simulink model "PID"  (R2018b)
settings: Solver=ode4  StartTime=0.0  StopTime=100  FixedStep=0.002  RelTol=1e-3
undefined symbols (not defined in the file): delta_mais, delta_menos, Kd, Ki, Km, Kp, tau
settings Model: Creator=pedro  LastModifiedBy=pedro
settings SFSimCC: SimUseLocalCustomCode=off
settings RTWCC: RTWUseLocalCustomCode=off
settings CodeAppCC: StateflowObjectComments=on

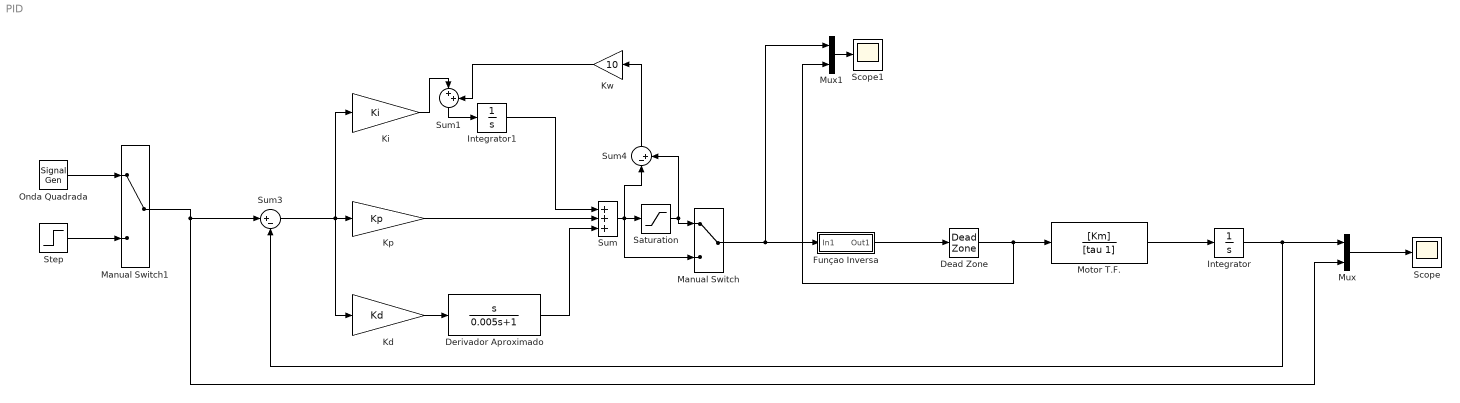
== system PID ==
  Dead Zone : DeadZone  LowerValue=-0.1154  UpperValue=0.2029  SaturateOnIntegerOverflow=on
  Derivador Aproximado : TransferFcn  Numerator=[1 0]  Denominator=[0.005 1]
  Funçao Inversa : Subsystem
  Integrator : Integrator
  Integrator1 : Integrator
  Kd : Gain  Gain=Kd
  Ki : Gain  Gain=Ki
  Kp : Gain  Gain=Kp
  Kw : Gain  Gain=10
  Manual Switch : ManualSwitch
  Manual Switch1 : ManualSwitch
  Motor T.F. : TransferFcn  Numerator=[Km]  Denominator=[tau 1]
  Mux : Mux  Inputs=2
  Mux1 : Mux  Inputs=2
  Onda Quadrada : SignalGenerator  WaveForm=square  Amplitude=20  Units=rad/sec
  Saturation : Saturate  UpperLimit=7.2  LowerLimit=-7.2
  Scope : Scope
  Scope1 : Scope
  Step : Step  SampleTime=0
  Sum : Sum  Inputs=|+|+|+|
  Sum1 : Sum  Inputs=|++
  Sum3 : Sum  Inputs=|+-
  Sum4 : Sum  Inputs=|-+
  wires:
  Motor T.F./1 -> Integrator/1
  Dead Zone/1 -> Mux1/2, Motor T.F./1
  Integrator/1 -> Mux/1, Sum3/2
  Sum3/1 -> Kp/1, Ki/1, Kd/1
  Kd/1 -> Derivador Aproximado/1
  Integrator1/1 -> Sum/1
  Kp/1 -> Sum/2
  Sum/1 -> Sum4/1, Manual Switch/2, Saturation/1
  Saturation/1 -> Sum4/2, Manual Switch/1
  Sum4/1 -> Kw/1
  Ki/1 -> Sum1/1
  Sum1/1 -> Integrator1/1
  Kw/1 -> Sum1/2
  Funçao Inversa/1(Out1) -> Dead Zone/1
  Mux/1 -> Scope/1
  Manual Switch1/1 -> Mux/2, Sum3/1
  Derivador Aproximado/1 -> Sum/3
  Manual Switch/1 -> Mux1/1, Funçao Inversa/1(In1)
  Step/1 -> Manual Switch1/2
  Onda Quadrada/1 -> Manual Switch1/1
  Mux1/1 -> Scope1/1

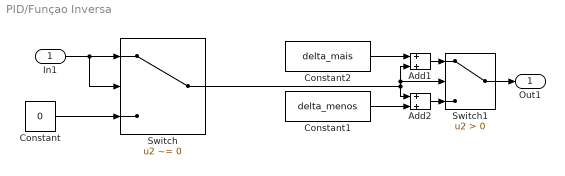
== system PID/Funçao Inversa ==
  In1 : Inport
  Add1 : Sum
  Add2 : Sum
  Constant : Constant  Value=0
  Constant1 : Constant  Value=delta_menos
  Constant2 : Constant  Value=delta_mais
  Switch : Switch  Criteria=u2 ~= 0
  Switch1 : Switch  Criteria=u2 > Threshold
  Out1 : Outport
  wires:
  Switch/1 -> Add1/2, Switch1/2, Add2/1
  Constant1/1 -> Add2/2
  In1/1 -> Switch/2, Switch/1
  Constant/1 -> Switch/3
  Switch1/1 -> Out1/1
  Add2/1 -> Switch1/3
  Add1/1 -> Switch1/1
  Constant2/1 -> Add1/1
